simulink library "DAQ_lib_HallPositionTorque"  (R2014b)
settings: Solver=ode45  StartTime=0.0  StopTime=10.0  RelTol=1e-3
undefined symbols (not defined in the file): A_lpf_velocity, ANOMALY_INIT, B1_lpf_velocity, B2_lpf_velocity, Calibration, EnableFT, EncoderAngleLimits, EncoderFiltSys, EncoderThreshold, FTCalibration, GearOffsets, IMUAngleLimits, IMUCommand, IMUThreshold, IMUTorsoOffsets, m_XR17D15x, MAX_ANOMALY, MedullaCommand, MicrostrainFiltSys, MODBUS_TIMEOUT, ResetDAQ, ResetYaw, sample_time, standard, STREAMING_TIMEOUT, TareFT, TorsoCOMOffsets, Ts, TsCAN, TsKVH, UseMicrostrainRate
libraries: xpcethercatlib x207, simulink x53, canmsglib x21, speedgoatlib x13, slrtlib x5, speedgoatlib_IO601 x5, dspswit3 x2, dspmtrx3 x2, xpcseriallib x1, SpeedgoatModified x1
(part 3 of 7)

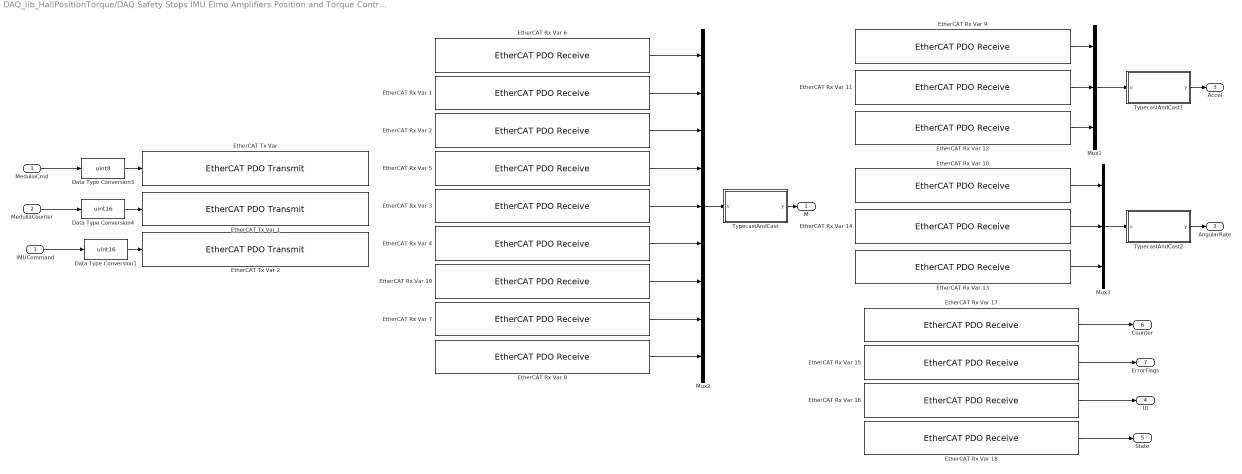
== system DAQ_lib_HallPositionTorque/DAQ Safety Stops IMU Elmo Amplifiers Position and Torque Control with Hall Sensors/DAQ/EtherCATNetwork/EtherCATRobotMicrostrain/IMU_Medulla ==
  MedullaCmd : Inport
  MedullaCounter : Inport  Port=2
  IMUCommand : Inport  Port=3
  Data Type Conversion1 : DataTypeConversion  OutDataTypeStr=uint16  RndMeth=Simplest
  Data Type Conversion3 : DataTypeConversion  OutDataTypeStr=uint8  RndMeth=Simplest
  Data Type Conversion4 : DataTypeConversion  OutDataTypeStr=uint16  RndMeth=Simplest
  EtherCAT Rx Var 1 : xpcethercatlib/EtherCAT PDO Receive  Priority=2  sig_name=Box 7 (ATRIAS 2.1 Microstrain IMU (Medulla 1.5)).M.M12  sig_offset=2784  sig_type=uint32  type_size=32  sig_dim=1  device_id=0  sample_time=0.000500
  EtherCAT Rx Var 10 : xpcethercatlib/EtherCAT PDO Receive  Priority=2  sig_name=Box 7 (ATRIAS 2.1 Microstrain IMU (Medulla 1.5)).Xaxes.XAngRate  sig_offset=2560  sig_type=uint32  type_size=32  sig_dim=1  device_id=0  sample_time=0.000500
  EtherCAT Rx Var 11 : xpcethercatlib/EtherCAT PDO Receive  Priority=2  sig_name=Box 7 (ATRIAS 2.1 Microstrain IMU (Medulla 1.5)).Yaxes.YAccel  sig_offset=2656  sig_type=uint32  type_size=32  sig_dim=1  device_id=0  sample_time=0.000500
  EtherCAT Rx Var 12 : xpcethercatlib/EtherCAT PDO Receive  Priority=2  sig_name=Box 7 (ATRIAS 2.1 Microstrain IMU (Medulla 1.5)).Zaxes.ZAccel  sig_offset=2720  sig_type=uint32  type_size=32  sig_dim=1  device_id=0  sample_time=0.000500
  EtherCAT Rx Var 13 : xpcethercatlib/EtherCAT PDO Receive  Priority=2  sig_name=Box 7 (ATRIAS 2.1 Microstrain IMU (Medulla 1.5)).Zaxes.ZAngRate  sig_offset=2688  sig_type=uint32  type_size=32  sig_dim=1  device_id=0  sample_time=0.000500
  EtherCAT Rx Var 14 : xpcethercatlib/EtherCAT PDO Receive  Priority=2  sig_name=Box 7 (ATRIAS 2.1 Microstrain IMU (Medulla 1.5)).Yaxes.YAngRate  sig_offset=2624  sig_type=uint32  type_size=32  sig_dim=1  device_id=0  sample_time=0.000500
  EtherCAT Rx Var 15 : xpcethercatlib/EtherCAT PDO Receive  Priority=2  sig_name=Box 7 (ATRIAS 2.1 Microstrain IMU (Medulla 1.5)).uController Status.Error Flags  sig_offset=2552  sig_type=uint8  type_size=8  sig_dim=1  device_id=0  sample_time=0.000500
  EtherCAT Rx Var 16 : xpcethercatlib/EtherCAT PDO Receive  Priority=2  sig_name=Box 7 (ATRIAS 2.1 Microstrain IMU (Medulla 1.5)).uController Status.ID  sig_offset=2528  sig_type=uint8  type_size=8  sig_dim=1  device_id=0  sample_time=0.000500
  EtherCAT Rx Var 17 : xpcethercatlib/EtherCAT PDO Receive  Priority=2  sig_name=Box 7 (ATRIAS 2.1 Microstrain IMU (Medulla 1.5)).uController Status.Counter  sig_offset=2544  sig_type=uint8  type_size=8  sig_dim=1  device_id=0  sample_time=0.000500
  EtherCAT Rx Var 18 : xpcethercatlib/EtherCAT PDO Receive  Priority=2  sig_name=Box 7 (ATRIAS 2.1 Microstrain IMU (Medulla 1.5)).uController Status.State  sig_offset=2536  sig_type=uint8  type_size=8  sig_dim=1  device_id=0  sample_time=0.000500
  EtherCAT Rx Var 19 : xpcethercatlib/EtherCAT PDO Receive  Priority=2  sig_name=Box 7 (ATRIAS 2.1 Microstrain IMU (Medulla 1.5)).M.M31  sig_offset=2944  sig_type=uint32  type_size=32  sig_dim=1  device_id=0  sample_time=0.000500
  EtherCAT Rx Var 2 : xpcethercatlib/EtherCAT PDO Receive  Priority=2  sig_name=Box 7 (ATRIAS 2.1 Microstrain IMU (Medulla 1.5)).M.M13  sig_offset=2816  sig_type=uint32  type_size=32  sig_dim=1  device_id=0  sample_time=0.000500
  EtherCAT Rx Var 3 : xpcethercatlib/EtherCAT PDO Receive  Priority=2  sig_name=Box 7 (ATRIAS 2.1 Microstrain IMU (Medulla 1.5)).M.M22  sig_offset=2880  sig_type=uint32  type_size=32  sig_dim=1  device_id=0  sample_time=0.000500
  EtherCAT Rx Var 4 : xpcethercatlib/EtherCAT PDO Receive  Priority=2  sig_name=Box 7 (ATRIAS 2.1 Microstrain IMU (Medulla 1.5)).M.M23  sig_offset=2912  sig_type=uint32  type_size=32  sig_dim=1  device_id=0  sample_time=0.000500
  EtherCAT Rx Var 5 : xpcethercatlib/EtherCAT PDO Receive  Priority=2  sig_name=Box 7 (ATRIAS 2.1 Microstrain IMU (Medulla 1.5)).M.M21  sig_offset=2848  sig_type=uint32  type_size=32  sig_dim=1  device_id=0  sample_time=0.000500
  EtherCAT Rx Var 6 : xpcethercatlib/EtherCAT PDO Receive  Priority=2  sig_name=Box 7 (ATRIAS 2.1 Microstrain IMU (Medulla 1.5)).M.M11  sig_offset=2752  sig_type=uint32  type_size=32  sig_dim=1  device_id=0  sample_time=0.000500
  EtherCAT Rx Var 7 : xpcethercatlib/EtherCAT PDO Receive  Priority=2  sig_name=Box 7 (ATRIAS 2.1 Microstrain IMU (Medulla 1.5)).M.M32  sig_offset=2976  sig_type=uint32  type_size=32  sig_dim=1  device_id=0  sample_time=0.000500
  EtherCAT Rx Var 8 : xpcethercatlib/EtherCAT PDO Receive  Priority=2  sig_name=Box 7 (ATRIAS 2.1 Microstrain IMU (Medulla 1.5)).M.M33  sig_offset=3008  sig_type=uint32  type_size=32  sig_dim=1  device_id=0  sample_time=0.000500
  EtherCAT Rx Var 9 : xpcethercatlib/EtherCAT PDO Receive  Priority=2  sig_name=Box 7 (ATRIAS 2.1 Microstrain IMU (Medulla 1.5)).Xaxes.XAccel  sig_offset=2592  sig_type=uint32  type_size=32  sig_dim=1  device_id=0  sample_time=0.000500
  "EtherCAT Tx Var " : xpcethercatlib/EtherCAT PDO Transmit   Priority=3  sig_name=Box 7 (ATRIAS 2.1 Microstrain IMU (Medulla 1.5)).uControllerInput.Command  sig_offset=2528  sig_type=uint8  type_size=8  sig_dim=1  device_id=0  sample_time=0.000500
  EtherCAT Tx Var 1 : xpcethercatlib/EtherCAT PDO Transmit   Priority=3  sig_name=Box 7 (ATRIAS 2.1 Microstrain IMU (Medulla 1.5)).uControllerInput.Counter  sig_offset=2536  sig_type=uint16  type_size=16  sig_dim=1  device_id=0  sample_time=0.000500
  EtherCAT Tx Var 2 : xpcethercatlib/EtherCAT PDO Transmit   Priority=3  sig_name=Box 7 (ATRIAS 2.1 Microstrain IMU (Medulla 1.5)).uControllerInput.IMU_cmd  sig_offset=2552  sig_type=uint16  type_size=16  sig_dim=1  device_id=0  sample_time=0.000500
  Mux1 : Mux  Inputs=3
  Mux2 : Mux  Inputs=9
  Mux3 : Mux  Inputs=3
  TypecastAndCast : MATLAB Function  TreatAsAtomicUnit=on
  TypecastAndCast1 : MATLAB Function  TreatAsAtomicUnit=on
  TypecastAndCast2 : MATLAB Function  TreatAsAtomicUnit=on
  M : Outport
  AngularRate : Outport  Port=2
  Accel : Outport  Port=3
  ID : Outport  Port=4
  State : Outport  Port=5
  Counter : Outport  Port=6
  ErrorFlags : Outport  Port=7
  wires:
  Data Type Conversion3/1 -> "EtherCAT Tx Var "/1
  Data Type Conversion4/1 -> EtherCAT Tx Var 1/1
  MedullaCmd/1 -> Data Type Conversion3/1
  MedullaCounter/1 -> Data Type Conversion4/1
  IMUCommand/1 -> Data Type Conversion1/1
  Data Type Conversion1/1 -> EtherCAT Tx Var 2/1
  EtherCAT Rx Var 17/1 -> Counter/1
  EtherCAT Rx Var 15/1 -> ErrorFlags/1
  EtherCAT Rx Var 16/1 -> ID/1
  EtherCAT Rx Var 18/1 -> State/1
  EtherCAT Rx Var 13/1 -> Mux3/3
  EtherCAT Rx Var 14/1 -> Mux3/2
  EtherCAT Rx Var 10/1 -> Mux3/1
  EtherCAT Rx Var 12/1 -> Mux1/3
  EtherCAT Rx Var 11/1 -> Mux1/2
  EtherCAT Rx Var 9/1 -> Mux1/1
  Mux1/1 -> TypecastAndCast1/1(u)
  Mux3/1 -> TypecastAndCast2/1(u)
  Mux2/1 -> TypecastAndCast/1(u)
  TypecastAndCast/1(y) -> M/1
  TypecastAndCast1/1(y) -> Accel/1
  TypecastAndCast2/1(y) -> AngularRate/1
  EtherCAT Rx Var 1/1 -> Mux2/2
  EtherCAT Rx Var 19/1 -> Mux2/7
  EtherCAT Rx Var 2/1 -> Mux2/3
  EtherCAT Rx Var 3/1 -> Mux2/5
  EtherCAT Rx Var 4/1 -> Mux2/6
  EtherCAT Rx Var 5/1 -> Mux2/4
  EtherCAT Rx Var 6/1 -> Mux2/1
  EtherCAT Rx Var 7/1 -> Mux2/8
  EtherCAT Rx Var 8/1 -> Mux2/9

== system DAQ_lib_HallPositionTorque/DAQ Safety Stops IMU Elmo Amplifiers Position and Torque Control with Hall Sensors/DAQ/EtherCATNetwork/EtherCATRobotMicrostrain/LegElmo_1L ==
  note: 1, 8 = Position Control
      | 3, 9 = Velocity Control
      | 4, 10 = Current Control
  MedullaCommand : Inport
  Mode of Operation : Inport  Port=2
  Desired Position : Inport  Port=3
  Desired Torque : Inport  Port=4
  Max Torque : Inport  Port=5
  Data Type Conversion{1..2,4,20,42,46} (6 alike) : DataTypeConversion  OutDataTypeStr=double
  Data Type Conversion5 : DataTypeConversion  OutDataTypeStr=int32
  EtherCATSubsystem : Subsystem
  MaxRatedCurrent : Constant  Value=48.47  OutDataTypeStr=double
  State Flow : Stateflow chart  TreatAsAtomicUnit=on
  Subsystem1 : Subsystem
  Subsystem10 : Subsystem
  Subsystem2 : Subsystem
  Subsystem3 : Subsystem
  Subsystem4 : Subsystem
  Subsystem5 : Subsystem
  Subsystem6 : Subsystem
  Subsystem7 : Subsystem
  Terminator : Terminator
  Actual Current : Outport
  Status Word : Outport  Port=2
  Actual Velocity : Outport  Port=3
  Mode of Operation Display : Outport  Port=4
  FaultDetected : Outport  Port=5
  Actual Position : Outport  Port=6
  Control Word Index : Outport  Port=7
  wires:
  Subsystem7/1(ScaledValue) -> EtherCATSubsystem/5(Max Torque)
  Max Torque/1 -> Subsystem7/1(ActualValue)
  [MaxRatedCurrent] -> Subsystem7/2(MaxRatedCurrent)
  Data Type Conversion20/1 -> Actual Current/1
  Data Type Conversion1/1 -> Actual Velocity/1
  Data Type Conversion46/1 -> Mode of Operation Display/1
  Subsystem2/1(SwitchOnDisabledMode) -> State Flow/1(SwitchOnDisabledMode)
  Subsystem3/1(EnabledMode) -> State Flow/2(EnabledMode)
  Subsystem4/1(ReadyToSwitchOnMode) -> State Flow/3(ReadyToSwitchOnMode)
  Subsystem5/1(FaultMode) -> State Flow/4(FaultMode)
  [MaxRatedCurrent] -> Subsystem6/2(MaxRatedCurrent)
  Subsystem6/1(ActualValue) -> Data Type Conversion20/1
  MaxRatedCurrent/1 -> [MaxRatedCurrent]
  State Flow/3(FaultDetected) -> FaultDetected/1
  MedullaCommand/1 -> State Flow/5(MedullaCommand)
  Data Type Conversion2/1 -> Subsystem6/1(ScaledValue)
  Subsystem1/1(ControlWord) -> EtherCATSubsystem/1(Control Word)
  Mode of Operation/1 -> EtherCATSubsystem/2(Mode of Operation)
  EtherCATSubsystem/5(Actual Torque) -> Data Type Conversion2/1
  Data Type Conversion4/1 -> Actual Position/1
  EtherCATSubsystem/2(Mode of Operation Display) -> Data Type Conversion46/1
  EtherCATSubsystem/1(Status Word) -> Subsystem5/1(StatusWord), Subsystem4/1(StatusWord), Subsystem3/1(StatusWord), Subsystem2/1(StatusWord), Data Type Conversion42/1
  Data Type Conversion42/1 -> Status Word/1
  Desired Torque/1 -> Subsystem10/1(ActualValue)
  [MaxRatedCurrent] -> Subsystem10/2(MaxRatedCurrent)
  Subsystem10/1(ScaledValue) -> EtherCATSubsystem/4(Target Torque)
  EtherCATSubsystem/3(Actual Position) -> Data Type Conversion4/1
  EtherCATSubsystem/4(Actual Velocity) -> Data Type Conversion1/1
  State Flow/2(Enable) -> Terminator/1
  Data Type Conversion5/1 -> EtherCATSubsystem/3(Target Position)
  Desired Position/1 -> Data Type Conversion5/1
  State Flow/1(ControlWordIndex) -> Control Word Index/1, Subsystem1/1(ControlWordIndex)

== system DAQ_lib_HallPositionTorque/DAQ Safety Stops IMU Elmo Amplifiers Position and Torque Control with Hall Sensors/DAQ/EtherCATNetwork/EtherCATRobotMicrostrain/LegElmo_1R ==
  note: 1, 8 = Position Control
      | 3, 9 = Velocity Control
      | 4, 10 = Current Control
  MedullaCommand : Inport
  Mode of Operation : Inport  Port=2
  Desired Position : Inport  Port=3
  Desired Torque : Inport  Port=4
  Max Torque : Inport  Port=5
  Data Type Conversion{1..2,4,20,42,46} (6 alike) : DataTypeConversion  OutDataTypeStr=double
  Data Type Conversion5 : DataTypeConversion  OutDataTypeStr=int32
  EtherCATSubsystem : Subsystem
  MaxRatedCurrent : Constant  Value=48.47  OutDataTypeStr=double
  State Flow : Stateflow chart  TreatAsAtomicUnit=on
  Subsystem1 : Subsystem
  Subsystem10 : Subsystem
  Subsystem2 : Subsystem
  Subsystem3 : Subsystem
  Subsystem4 : Subsystem
  Subsystem5 : Subsystem
  Subsystem6 : Subsystem
  Subsystem7 : Subsystem
  Terminator : Terminator
  Actual Current : Outport
  Status Word : Outport  Port=2
  Actual Velocity : Outport  Port=3
  Mode of Operation Display : Outport  Port=4
  FaultDetected : Outport  Port=5
  Actual Position : Outport  Port=6
  Control Word Index : Outport  Port=7
  wires:
  Subsystem7/1(ScaledValue) -> EtherCATSubsystem/5(Max Torque)
  Max Torque/1 -> Subsystem7/1(ActualValue)
  [MaxRatedCurrent] -> Subsystem7/2(MaxRatedCurrent)
  Data Type Conversion20/1 -> Actual Current/1
  Data Type Conversion1/1 -> Actual Velocity/1
  Data Type Conversion46/1 -> Mode of Operation Display/1
  Subsystem2/1(SwitchOnDisabledMode) -> State Flow/1(SwitchOnDisabledMode)
  Subsystem3/1(EnabledMode) -> State Flow/2(EnabledMode)
  Subsystem4/1(ReadyToSwitchOnMode) -> State Flow/3(ReadyToSwitchOnMode)
  Subsystem5/1(FaultMode) -> State Flow/4(FaultMode)
  [MaxRatedCurrent] -> Subsystem6/2(MaxRatedCurrent)
  Subsystem6/1(ActualValue) -> Data Type Conversion20/1
  MaxRatedCurrent/1 -> [MaxRatedCurrent]
  State Flow/3(FaultDetected) -> FaultDetected/1
  MedullaCommand/1 -> State Flow/5(MedullaCommand)
  Data Type Conversion2/1 -> Subsystem6/1(ScaledValue)
  Subsystem1/1(ControlWord) -> EtherCATSubsystem/1(Control Word)
  Mode of Operation/1 -> EtherCATSubsystem/2(Mode of Operation)
  EtherCATSubsystem/5(Actual Torque) -> Data Type Conversion2/1
  Data Type Conversion4/1 -> Actual Position/1
  EtherCATSubsystem/2(Mode of Operation Display) -> Data Type Conversion46/1
  EtherCATSubsystem/1(Status Word) -> Subsystem5/1(StatusWord), Subsystem4/1(StatusWord), Subsystem3/1(StatusWord), Subsystem2/1(StatusWord), Data Type Conversion42/1
  Data Type Conversion42/1 -> Status Word/1
  Desired Torque/1 -> Subsystem10/1(ActualValue)
  [MaxRatedCurrent] -> Subsystem10/2(MaxRatedCurrent)
  Subsystem10/1(ScaledValue) -> EtherCATSubsystem/4(Target Torque)
  EtherCATSubsystem/3(Actual Position) -> Data Type Conversion4/1
  EtherCATSubsystem/4(Actual Velocity) -> Data Type Conversion1/1
  State Flow/2(Enable) -> Terminator/1
  Data Type Conversion5/1 -> EtherCATSubsystem/3(Target Position)
  Desired Position/1 -> Data Type Conversion5/1
  State Flow/1(ControlWordIndex) -> Control Word Index/1, Subsystem1/1(ControlWordIndex)

== system DAQ_lib_HallPositionTorque/DAQ Safety Stops IMU Elmo Amplifiers Position and Torque Control with Hall Sensors/DAQ/EtherCATNetwork/EtherCATRobotMicrostrain/LegElmo_2L ==
  note: 1, 8 = Position Control
      | 3, 9 = Velocity Control
      | 4, 10 = Current Control
  MedullaCommand : Inport
  Mode of Operation : Inport  Port=2
  Desired Position : Inport  Port=3
  Desired Torque : Inport  Port=4
  Max Torque : Inport  Port=5
  Data Type Conversion{1..2,4,20,42,46} (6 alike) : DataTypeConversion  OutDataTypeStr=double
  Data Type Conversion5 : DataTypeConversion  OutDataTypeStr=int32
  EtherCATSubsystem : Subsystem
  MaxRatedCurrent : Constant  Value=48.47  OutDataTypeStr=double
  State Flow : Stateflow chart  TreatAsAtomicUnit=on
  Subsystem1 : Subsystem
  Subsystem10 : Subsystem
  Subsystem2 : Subsystem
  Subsystem3 : Subsystem
  Subsystem4 : Subsystem
  Subsystem5 : Subsystem
  Subsystem6 : Subsystem
  Subsystem7 : Subsystem
  Terminator : Terminator
  Actual Current : Outport
  Status Word : Outport  Port=2
  Actual Velocity : Outport  Port=3
  Mode of Operation Display : Outport  Port=4
  FaultDetected : Outport  Port=5
  Actual Position : Outport  Port=6
  Control Word Index : Outport  Port=7
  wires:
  Subsystem7/1(ScaledValue) -> EtherCATSubsystem/5(Max Torque)
  Max Torque/1 -> Subsystem7/1(ActualValue)
  [MaxRatedCurrent] -> Subsystem7/2(MaxRatedCurrent)
  Data Type Conversion20/1 -> Actual Current/1
  Data Type Conversion1/1 -> Actual Velocity/1
  Data Type Conversion46/1 -> Mode of Operation Display/1
  Subsystem2/1(SwitchOnDisabledMode) -> State Flow/1(SwitchOnDisabledMode)
  Subsystem3/1(EnabledMode) -> State Flow/2(EnabledMode)
  Subsystem4/1(ReadyToSwitchOnMode) -> State Flow/3(ReadyToSwitchOnMode)
  Subsystem5/1(FaultMode) -> State Flow/4(FaultMode)
  [MaxRatedCurrent] -> Subsystem6/2(MaxRatedCurrent)
  Subsystem6/1(ActualValue) -> Data Type Conversion20/1
  MaxRatedCurrent/1 -> [MaxRatedCurrent]
  State Flow/3(FaultDetected) -> FaultDetected/1
  MedullaCommand/1 -> State Flow/5(MedullaCommand)
  Data Type Conversion2/1 -> Subsystem6/1(ScaledValue)
  Subsystem1/1(ControlWord) -> EtherCATSubsystem/1(Control Word)
  Mode of Operation/1 -> EtherCATSubsystem/2(Mode of Operation)
  EtherCATSubsystem/5(Actual Torque) -> Data Type Conversion2/1
  Data Type Conversion4/1 -> Actual Position/1
  EtherCATSubsystem/2(Mode of Operation Display) -> Data Type Conversion46/1
  EtherCATSubsystem/1(Status Word) -> Subsystem5/1(StatusWord), Subsystem4/1(StatusWord), Subsystem3/1(StatusWord), Subsystem2/1(StatusWord), Data Type Conversion42/1
  Data Type Conversion42/1 -> Status Word/1
  Desired Torque/1 -> Subsystem10/1(ActualValue)
  [MaxRatedCurrent] -> Subsystem10/2(MaxRatedCurrent)
  Subsystem10/1(ScaledValue) -> EtherCATSubsystem/4(Target Torque)
  EtherCATSubsystem/3(Actual Position) -> Data Type Conversion4/1
  EtherCATSubsystem/4(Actual Velocity) -> Data Type Conversion1/1
  State Flow/2(Enable) -> Terminator/1
  Data Type Conversion5/1 -> EtherCATSubsystem/3(Target Position)
  Desired Position/1 -> Data Type Conversion5/1
  State Flow/1(ControlWordIndex) -> Control Word Index/1, Subsystem1/1(ControlWordIndex)

== system DAQ_lib_HallPositionTorque/DAQ Safety Stops IMU Elmo Amplifiers Position and Torque Control with Hall Sensors/DAQ/EtherCATNetwork/EtherCATRobotMicrostrain/LegElmo_2R ==
  note: 1, 8 = Position Control
      | 3, 9 = Velocity Control
      | 4, 10 = Current Control
  MedullaCommand : Inport
  Mode of Operation : Inport  Port=2
  Desired Position : Inport  Port=3
  Desired Torque : Inport  Port=4
  Max Torque : Inport  Port=5
  Data Type Conversion{1..2,4,20,42,46} (6 alike) : DataTypeConversion  OutDataTypeStr=double
  Data Type Conversion5 : DataTypeConversion  OutDataTypeStr=int32
  EtherCATSubsystem : Subsystem
  MaxRatedCurrent : Constant  Value=48.47  OutDataTypeStr=double
  State Flow : Stateflow chart  TreatAsAtomicUnit=on
  Subsystem1 : Subsystem
  Subsystem10 : Subsystem
  Subsystem2 : Subsystem
  Subsystem3 : Subsystem
  Subsystem4 : Subsystem
  Subsystem5 : Subsystem
  Subsystem6 : Subsystem
  Subsystem7 : Subsystem
  Terminator : Terminator
  Actual Current : Outport
  Status Word : Outport  Port=2
  Actual Velocity : Outport  Port=3
  Mode of Operation Display : Outport  Port=4
  FaultDetected : Outport  Port=5
  Actual Position : Outport  Port=6
  Control Word Index : Outport  Port=7
  wires:
  Subsystem7/1(ScaledValue) -> EtherCATSubsystem/5(Max Torque)
  Max Torque/1 -> Subsystem7/1(ActualValue)
  [MaxRatedCurrent] -> Subsystem7/2(MaxRatedCurrent)
  Data Type Conversion20/1 -> Actual Current/1
  Data Type Conversion1/1 -> Actual Velocity/1
  Data Type Conversion46/1 -> Mode of Operation Display/1
  Subsystem2/1(SwitchOnDisabledMode) -> State Flow/1(SwitchOnDisabledMode)
  Subsystem3/1(EnabledMode) -> State Flow/2(EnabledMode)
  Subsystem4/1(ReadyToSwitchOnMode) -> State Flow/3(ReadyToSwitchOnMode)
  Subsystem5/1(FaultMode) -> State Flow/4(FaultMode)
  [MaxRatedCurrent] -> Subsystem6/2(MaxRatedCurrent)
  Subsystem6/1(ActualValue) -> Data Type Conversion20/1
  MaxRatedCurrent/1 -> [MaxRatedCurrent]
  State Flow/3(FaultDetected) -> FaultDetected/1
  MedullaCommand/1 -> State Flow/5(MedullaCommand)
  Data Type Conversion2/1 -> Subsystem6/1(ScaledValue)
  Subsystem1/1(ControlWord) -> EtherCATSubsystem/1(Control Word)
  Mode of Operation/1 -> EtherCATSubsystem/2(Mode of Operation)
  EtherCATSubsystem/5(Actual Torque) -> Data Type Conversion2/1
  Data Type Conversion4/1 -> Actual Position/1
  EtherCATSubsystem/2(Mode of Operation Display) -> Data Type Conversion46/1
  EtherCATSubsystem/1(Status Word) -> Subsystem5/1(StatusWord), Subsystem4/1(StatusWord), Subsystem3/1(StatusWord), Subsystem2/1(StatusWord), Data Type Conversion42/1
  Data Type Conversion42/1 -> Status Word/1
  Desired Torque/1 -> Subsystem10/1(ActualValue)
  [MaxRatedCurrent] -> Subsystem10/2(MaxRatedCurrent)
  Subsystem10/1(ScaledValue) -> EtherCATSubsystem/4(Target Torque)
  EtherCATSubsystem/3(Actual Position) -> Data Type Conversion4/1
  EtherCATSubsystem/4(Actual Velocity) -> Data Type Conversion1/1
  State Flow/2(Enable) -> Terminator/1
  Data Type Conversion5/1 -> EtherCATSubsystem/3(Target Position)
  Desired Position/1 -> Data Type Conversion5/1
  State Flow/1(ControlWordIndex) -> Control Word Index/1, Subsystem1/1(ControlWordIndex)

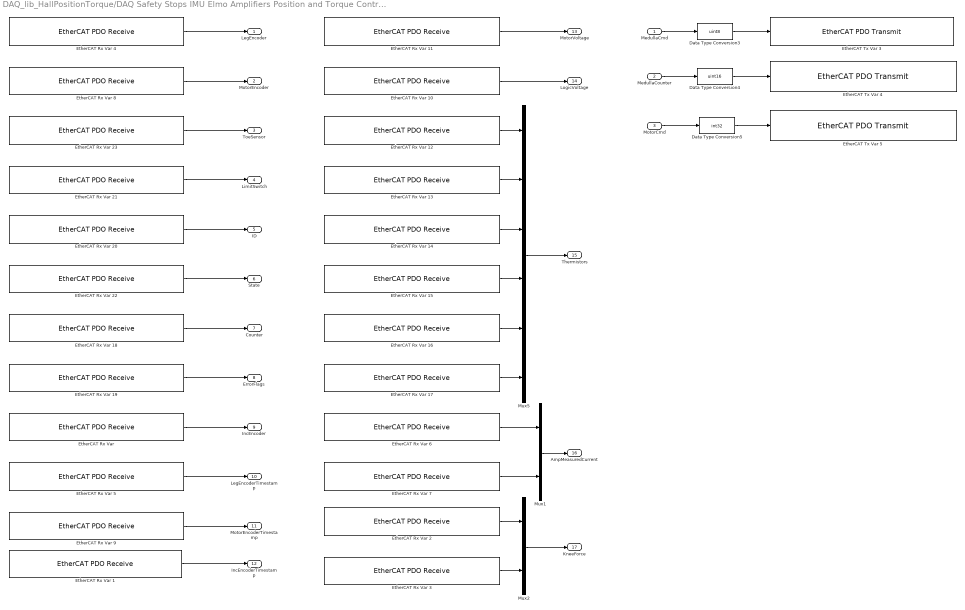
== system DAQ_lib_HallPositionTorque/DAQ Safety Stops IMU Elmo Amplifiers Position and Torque Control with Hall Sensors/DAQ/EtherCATNetwork/EtherCATRobotMicrostrain/LegMedulla_1L ==
  MedullaCmd : Inport
  MedullaCounter : Inport  Port=2
  MotorCmd : Inport  Port=3
  Data Type Conversion3 : DataTypeConversion  OutDataTypeStr=uint8  RndMeth=Simplest
  Data Type Conversion4 : DataTypeConversion  OutDataTypeStr=uint16  RndMeth=Simplest
  Data Type Conversion5 : DataTypeConversion  OutDataTypeStr=int32  RndMeth=Simplest
  "EtherCAT Rx Var " : xpcethercatlib/EtherCAT PDO Receive  Priority=2  sig_name=Box 1 (ATRIAS 2.1 Leg (Medulla 1.5)).Incremental Encoder.Incremental Encoder  sig_offset=744  sig_type=uint16  type_size=16  sig_dim=1  device_id=0  sample_time=0.000500
  EtherCAT Rx Var 1 : xpcethercatlib/EtherCAT PDO Receive  Priority=2  sig_name=Box 1 (ATRIAS 2.1 Leg (Medulla 1.5)).Incremental Encoder.Incremental Encoder Timestamp  sig_offset=760  sig_type=uint16  type_size=16  sig_dim=1  device_id=0  sample_time=0.000500
  EtherCAT Rx Var 10 : xpcethercatlib/EtherCAT PDO Receive  Priority=2  sig_name=Box 1 (ATRIAS 2.1 Leg (Medulla 1.5)).Power.Logic Voltage  sig_offset=792  sig_type=uint16  type_size=16  sig_dim=1  device_id=0  sample_time=0.000500
  EtherCAT Rx Var 11 : xpcethercatlib/EtherCAT PDO Receive  Priority=2  sig_name=Box 1 (ATRIAS 2.1 Leg (Medulla 1.5)).Power.Motor Voltage  sig_offset=776  sig_type=uint16  type_size=16  sig_dim=1  device_id=0  sample_time=0.000500
  EtherCAT Rx Var 12 : xpcethercatlib/EtherCAT PDO Receive  Priority=2  sig_name=Box 1 (ATRIAS 2.1 Leg (Medulla 1.5)).Thermistors.Thermistor 0  sig_offset=808  sig_type=uint16  type_size=16  sig_dim=1  device_id=0  sample_time=0.000500
  EtherCAT Rx Var 13 : xpcethercatlib/EtherCAT PDO Receive  Priority=2  sig_name=Box 1 (ATRIAS 2.1 Leg (Medulla 1.5)).Thermistors.Thermistor 1  sig_offset=824  sig_type=uint16  type_size=16  sig_dim=1  device_id=0  sample_time=0.000500
  EtherCAT Rx Var 14 : xpcethercatlib/EtherCAT PDO Receive  Priority=2  sig_name=Box 1 (ATRIAS 2.1 Leg (Medulla 1.5)).Thermistors.Thermistor 2  sig_offset=840  sig_type=uint16  type_size=16  sig_dim=1  device_id=0  sample_time=0.000500
  EtherCAT Rx Var 15 : xpcethercatlib/EtherCAT PDO Receive  Priority=2  sig_name=Box 1 (ATRIAS 2.1 Leg (Medulla 1.5)).Thermistors.Thermistor 3  sig_offset=856  sig_type=uint16  type_size=16  sig_dim=1  device_id=0  sample_time=0.000500
  EtherCAT Rx Var 16 : xpcethercatlib/EtherCAT PDO Receive  Priority=2  sig_name=Box 1 (ATRIAS 2.1 Leg (Medulla 1.5)).Thermistors.Thermistor 4  sig_offset=872  sig_type=uint16  type_size=16  sig_dim=1  device_id=0  sample_time=0.000500
  EtherCAT Rx Var 17 : xpcethercatlib/EtherCAT PDO Receive  Priority=2  sig_name=Box 1 (ATRIAS 2.1 Leg (Medulla 1.5)).Thermistors.Thermistor 5  sig_offset=888  sig_type=uint16  type_size=16  sig_dim=1  device_id=0  sample_time=0.000500
  EtherCAT Rx Var 18 : xpcethercatlib/EtherCAT PDO Receive  Priority=2  sig_name=Box 1 (ATRIAS 2.1 Leg (Medulla 1.5)).uController Status.Counter  sig_offset=608  sig_type=uint8  type_size=8  sig_dim=1  device_id=0  sample_time=0.000500
  EtherCAT Rx Var 19 : xpcethercatlib/EtherCAT PDO Receive  Priority=2  sig_name=Box 1 (ATRIAS 2.1 Leg (Medulla 1.5)).uController Status.Error Flags  sig_offset=616  sig_type=uint8  type_size=8  sig_dim=1  device_id=0  sample_time=0.000500
  EtherCAT Rx Var 2 : xpcethercatlib/EtherCAT PDO Receive  Priority=2  sig_name=Box 1 (ATRIAS 2.1 Leg (Medulla 1.5)).Knee Force.Knee Force 1  sig_offset=936  sig_type=uint16  type_size=16  sig_dim=1  device_id=0  sample_time=0.000500
  EtherCAT Rx Var 20 : xpcethercatlib/EtherCAT PDO Receive  Priority=2  sig_name=Box 1 (ATRIAS 2.1 Leg (Medulla 1.5)).uController Status.ID  sig_offset=592  sig_type=uint8  type_size=8  sig_dim=1  device_id=0  sample_time=0.000500
  EtherCAT Rx Var 21 : xpcethercatlib/EtherCAT PDO Receive  Priority=2  sig_name=Box 1 (ATRIAS 2.1 Leg (Medulla 1.5)).uController Status.Limit Switch  sig_offset=624  sig_type=uint8  type_size=8  sig_dim=1  device_id=0  sample_time=0.000500
  EtherCAT Rx Var 22 : xpcethercatlib/EtherCAT PDO Receive  Priority=2  sig_name=Box 1 (ATRIAS 2.1 Leg (Medulla 1.5)).uController Status.State  sig_offset=600  sig_type=uint8  type_size=8  sig_dim=1  device_id=0  sample_time=0.000500
  EtherCAT Rx Var 23 : xpcethercatlib/EtherCAT PDO Receive  Priority=2  sig_name=Box 1 (ATRIAS 2.1 Leg (Medulla 1.5)).uController Status.Toe Sensor  sig_offset=632  sig_type=uint16  type_size=16  sig_dim=1  device_id=0  sample_time=0.000500
  EtherCAT Rx Var 3 : xpcethercatlib/EtherCAT PDO Receive  Priority=2  sig_name=Box 1 (ATRIAS 2.1 Leg (Medulla 1.5)).Knee Force.Knee Force 2  sig_offset=952  sig_type=uint16  type_size=16  sig_dim=1  device_id=0  sample_time=0.000500
  EtherCAT Rx Var 4 : xpcethercatlib/EtherCAT PDO Receive  Priority=2  sig_name=Box 1 (ATRIAS 2.1 Leg (Medulla 1.5)).Leg Encoder.Leg Encoder  sig_offset=696  sig_type=uint32  type_size=32  sig_dim=1  device_id=0  sample_time=0.000500
  EtherCAT Rx Var 5 : xpcethercatlib/EtherCAT PDO Receive  Priority=2  sig_name=Box 1 (ATRIAS 2.1 Leg (Medulla 1.5)).Leg Encoder.Leg Encoder Timestamp  sig_offset=728  sig_type=uint16  type_size=16  sig_dim=1  device_id=0  sample_time=0.000500
  EtherCAT Rx Var 6 : xpcethercatlib/EtherCAT PDO Receive  Priority=2  sig_name=Box 1 (ATRIAS 2.1 Leg (Medulla 1.5)).Measured Current.Amp 1 Measured Current  sig_offset=904  sig_type=int16  type_size=16  sig_dim=1  device_id=0  sample_time=0.000500
  EtherCAT Rx Var 7 : xpcethercatlib/EtherCAT PDO Receive  Priority=2  sig_name=Box 1 (ATRIAS 2.1 Leg (Medulla 1.5)).Measured Current.Amp 2 Measured Current  sig_offset=920  sig_type=int16  type_size=16  sig_dim=1  device_id=0  sample_time=0.000500
  EtherCAT Rx Var 8 : xpcethercatlib/EtherCAT PDO Receive  Priority=2  sig_name=Box 1 (ATRIAS 2.1 Leg (Medulla 1.5)).Motor Encoder.Motor Encoder  sig_offset=648  sig_type=uint32  type_size=32  sig_dim=1  device_id=0  sample_time=0.000500
  EtherCAT Rx Var 9 : xpcethercatlib/EtherCAT PDO Receive  Priority=2  sig_name=Box 1 (ATRIAS 2.1 Leg (Medulla 1.5)).Motor Encoder.Motor Encoder Timestamp  sig_offset=680  sig_type=uint16  type_size=16  sig_dim=1  device_id=0  sample_time=0.000500
  EtherCAT Tx Var 3 : xpcethercatlib/EtherCAT PDO Transmit   Priority=3  sig_name=Box 1 (ATRIAS 2.1 Leg (Medulla 1.5)).uControllerInput.Command  sig_offset=592  sig_type=uint8  type_size=8  sig_dim=1  device_id=0  sample_time=0.000500
  EtherCAT Tx Var 4 : xpcethercatlib/EtherCAT PDO Transmit   Priority=3  sig_name=Box 1 (ATRIAS 2.1 Leg (Medulla 1.5)).uControllerInput.Counter  sig_offset=600  sig_type=uint16  type_size=16  sig_dim=1  device_id=0  sample_time=0.000500
  EtherCAT Tx Var 5 : xpcethercatlib/EtherCAT PDO Transmit   Priority=3  sig_name=Box 1 (ATRIAS 2.1 Leg (Medulla 1.5)).uControllerInput.Motor Current  sig_offset=616  sig_type=int32  type_size=32  sig_dim=1  device_id=0  sample_time=0.000500
  Mux1 : Mux  Inputs=2
  Mux2 : Mux  Inputs=2
  Mux5 : Mux  Inputs=6
  LegEncoder : Outport
  MotorEncoder : Outport  Port=2
  ToeSensor : Outport  Port=3
  LimitSwitch : Outport  Port=4
  ID : Outport  Port=5
  State : Outport  Port=6
  Counter : Outport  Port=7
  ErrorFlags : Outport  Port=8
  IncEncoder : Outport  Port=9
  LegEncoderTimestamp : Outport  Port=10
  MotorEncoderTimestamp : Outport  Port=11
  IncEncoderTimestamp : Outport  Port=12
  MotorVoltage : Outport  Port=13
  LogicVoltage : Outport  Port=14
  Thermistors : Outport  Port=15
  AmpMeasuredCurrent : Outport  Port=16
  KneeForce : Outport  Port=17
  wires:
  Data Type Conversion3/1 -> EtherCAT Tx Var 3/1
  Data Type Conversion4/1 -> EtherCAT Tx Var 4/1
  Data Type Conversion5/1 -> EtherCAT Tx Var 5/1
  "EtherCAT Rx Var "/1 -> IncEncoder/1
  EtherCAT Rx Var 1/1 -> IncEncoderTimestamp/1
  EtherCAT Rx Var 2/1 -> Mux2/1
  EtherCAT Rx Var 4/1 -> LegEncoder/1
  EtherCAT Rx Var 5/1 -> LegEncoderTimestamp/1
  EtherCAT Rx Var 6/1 -> Mux1/1
  EtherCAT Rx Var 8/1 -> MotorEncoder/1
  EtherCAT Rx Var 9/1 -> MotorEncoderTimestamp/1
  EtherCAT Rx Var 10/1 -> LogicVoltage/1
  EtherCAT Rx Var 11/1 -> MotorVoltage/1
  EtherCAT Rx Var 13/1 -> Mux5/2
  EtherCAT Rx Var 14/1 -> Mux5/3
  EtherCAT Rx Var 15/1 -> Mux5/4
  EtherCAT Rx Var 16/1 -> Mux5/5
  EtherCAT Rx Var 17/1 -> Mux5/6
  EtherCAT Rx Var 18/1 -> Counter/1
  EtherCAT Rx Var 19/1 -> ErrorFlags/1
  EtherCAT Rx Var 20/1 -> ID/1
  EtherCAT Rx Var 21/1 -> LimitSwitch/1
  EtherCAT Rx Var 22/1 -> State/1
  EtherCAT Rx Var 23/1 -> ToeSensor/1
  MedullaCmd/1 -> Data Type Conversion3/1
  MedullaCounter/1 -> Data Type Conversion4/1
  MotorCmd/1 -> Data Type Conversion5/1
  EtherCAT Rx Var 12/1 -> Mux5/1
  Mux5/1 -> Thermistors/1
  Mux1/1 -> AmpMeasuredCurrent/1
  EtherCAT Rx Var 7/1 -> Mux1/2
  EtherCAT Rx Var 3/1 -> Mux2/2
  Mux2/1 -> KneeForce/1

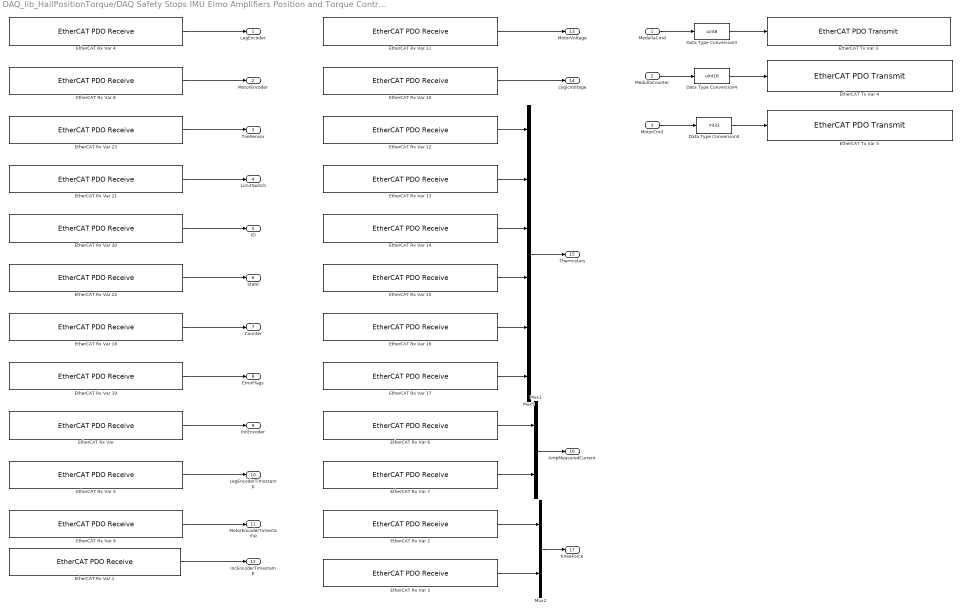
== system DAQ_lib_HallPositionTorque/DAQ Safety Stops IMU Elmo Amplifiers Position and Torque Control with Hall Sensors/DAQ/EtherCATNetwork/EtherCATRobotMicrostrain/LegMedulla_1R ==
  MedullaCmd : Inport
  MedullaCounter : Inport  Port=2
  MotorCmd : Inport  Port=3
  Data Type Conversion3 : DataTypeConversion  OutDataTypeStr=uint8  RndMeth=Simplest
  Data Type Conversion4 : DataTypeConversion  OutDataTypeStr=uint16  RndMeth=Simplest
  Data Type Conversion5 : DataTypeConversion  OutDataTypeStr=int32  RndMeth=Simplest
  "EtherCAT Rx Var " : xpcethercatlib/EtherCAT PDO Receive  Priority=2  sig_name=Box 3 (ATRIAS 2.1 Leg (Medulla 1.5)).Incremental Encoder.Incremental Encoder  sig_offset=1496  sig_type=uint16  type_size=16  sig_dim=1  device_id=0  sample_time=0.000500
  EtherCAT Rx Var 1 : xpcethercatlib/EtherCAT PDO Receive  Priority=2  sig_name=Box 3 (ATRIAS 2.1 Leg (Medulla 1.5)).Incremental Encoder.Incremental Encoder Timestamp  sig_offset=1512  sig_type=uint16  type_size=16  sig_dim=1  device_id=0  sample_time=0.000500
  EtherCAT Rx Var 10 : xpcethercatlib/EtherCAT PDO Receive  Priority=2  sig_name=Box 3 (ATRIAS 2.1 Leg (Medulla 1.5)).Power.Logic Voltage  sig_offset=1544  sig_type=uint16  type_size=16  sig_dim=1  device_id=0  sample_time=0.000500
  EtherCAT Rx Var 11 : xpcethercatlib/EtherCAT PDO Receive  Priority=2  sig_name=Box 3 (ATRIAS 2.1 Leg (Medulla 1.5)).Power.Motor Voltage  sig_offset=1528  sig_type=uint16  type_size=16  sig_dim=1  device_id=0  sample_time=0.000500
  EtherCAT Rx Var 12 : xpcethercatlib/EtherCAT PDO Receive  Priority=2  sig_name=Box 3 (ATRIAS 2.1 Leg (Medulla 1.5)).Thermistors.Thermistor 0  sig_offset=1560  sig_type=uint16  type_size=16  sig_dim=1  device_id=0  sample_time=0.000500
  EtherCAT Rx Var 13 : xpcethercatlib/EtherCAT PDO Receive  Priority=2  sig_name=Box 3 (ATRIAS 2.1 Leg (Medulla 1.5)).Thermistors.Thermistor 1  sig_offset=1576  sig_type=uint16  type_size=16  sig_dim=1  device_id=0  sample_time=0.000500
  EtherCAT Rx Var 14 : xpcethercatlib/EtherCAT PDO Receive  Priority=2  sig_name=Box 3 (ATRIAS 2.1 Leg (Medulla 1.5)).Thermistors.Thermistor 2  sig_offset=1592  sig_type=uint16  type_size=16  sig_dim=1  device_id=0  sample_time=0.000500
  EtherCAT Rx Var 15 : xpcethercatlib/EtherCAT PDO Receive  Priority=2  sig_name=Box 3 (ATRIAS 2.1 Leg (Medulla 1.5)).Thermistors.Thermistor 3  sig_offset=1608  sig_type=uint16  type_size=16  sig_dim=1  device_id=0  sample_time=0.000500
  EtherCAT Rx Var 16 : xpcethercatlib/EtherCAT PDO Receive  Priority=2  sig_name=Box 3 (ATRIAS 2.1 Leg (Medulla 1.5)).Thermistors.Thermistor 4  sig_offset=1624  sig_type=uint16  type_size=16  sig_dim=1  device_id=0  sample_time=0.000500
  EtherCAT Rx Var 17 : xpcethercatlib/EtherCAT PDO Receive  Priority=2  sig_name=Box 3 (ATRIAS 2.1 Leg (Medulla 1.5)).Thermistors.Thermistor 5  sig_offset=1640  sig_type=uint16  type_size=16  sig_dim=1  device_id=0  sample_time=0.000500
  EtherCAT Rx Var 18 : xpcethercatlib/EtherCAT PDO Receive  Priority=2  sig_name=Box 3 (ATRIAS 2.1 Leg (Medulla 1.5)).uController Status.Counter  sig_offset=1360  sig_type=uint8  type_size=8  sig_dim=1  device_id=0  sample_time=0.000500
  EtherCAT Rx Var 19 : xpcethercatlib/EtherCAT PDO Receive  Priority=2  sig_name=Box 3 (ATRIAS 2.1 Leg (Medulla 1.5)).uController Status.Error Flags  sig_offset=1368  sig_type=uint8  type_size=8  sig_dim=1  device_id=0  sample_time=0.000500
  EtherCAT Rx Var 2 : xpcethercatlib/EtherCAT PDO Receive  Priority=2  sig_name=Box 3 (ATRIAS 2.1 Leg (Medulla 1.5)).Knee Force.Knee Force 1  sig_offset=1688  sig_type=uint16  type_size=16  sig_dim=1  device_id=0  sample_time=0.000500
  EtherCAT Rx Var 20 : xpcethercatlib/EtherCAT PDO Receive  Priority=2  sig_name=Box 3 (ATRIAS 2.1 Leg (Medulla 1.5)).uController Status.ID  sig_offset=1344  sig_type=uint8  type_size=8  sig_dim=1  device_id=0  sample_time=0.000500
  EtherCAT Rx Var 21 : xpcethercatlib/EtherCAT PDO Receive  Priority=2  sig_name=Box 3 (ATRIAS 2.1 Leg (Medulla 1.5)).uController Status.Limit Switch  sig_offset=1376  sig_type=uint8  type_size=8  sig_dim=1  device_id=0  sample_time=0.000500
  EtherCAT Rx Var 22 : xpcethercatlib/EtherCAT PDO Receive  Priority=2  sig_name=Box 3 (ATRIAS 2.1 Leg (Medulla 1.5)).uController Status.State  sig_offset=1352  sig_type=uint8  type_size=8  sig_dim=1  device_id=0  sample_time=0.000500
  EtherCAT Rx Var 23 : xpcethercatlib/EtherCAT PDO Receive  Priority=2  sig_name=Box 3 (ATRIAS 2.1 Leg (Medulla 1.5)).uController Status.Toe Sensor  sig_offset=1384  sig_type=uint16  type_size=16  sig_dim=1  device_id=0  sample_time=0.000500
  EtherCAT Rx Var 3 : xpcethercatlib/EtherCAT PDO Receive  Priority=2  sig_name=Box 3 (ATRIAS 2.1 Leg (Medulla 1.5)).Knee Force.Knee Force 2  sig_offset=1704  sig_type=uint16  type_size=16  sig_dim=1  device_id=0  sample_time=0.000500
  EtherCAT Rx Var 4 : xpcethercatlib/EtherCAT PDO Receive  Priority=2  sig_name=Box 3 (ATRIAS 2.1 Leg (Medulla 1.5)).Leg Encoder.Leg Encoder  sig_offset=1448  sig_type=uint32  type_size=32  sig_dim=1  device_id=0  sample_time=0.000500
  EtherCAT Rx Var 5 : xpcethercatlib/EtherCAT PDO Receive  Priority=2  sig_name=Box 3 (ATRIAS 2.1 Leg (Medulla 1.5)).Leg Encoder.Leg Encoder Timestamp  sig_offset=1480  sig_type=uint16  type_size=16  sig_dim=1  device_id=0  sample_time=0.000500
  EtherCAT Rx Var 6 : xpcethercatlib/EtherCAT PDO Receive  Priority=2  sig_name=Box 3 (ATRIAS 2.1 Leg (Medulla 1.5)).Measured Current.Amp 1 Measured Current  sig_offset=1656  sig_type=int16  type_size=16  sig_dim=1  device_id=0  sample_time=0.000500
  EtherCAT Rx Var 7 : xpcethercatlib/EtherCAT PDO Receive  Priority=2  sig_name=Box 3 (ATRIAS 2.1 Leg (Medulla 1.5)).Measured Current.Amp 2 Measured Current  sig_offset=1672  sig_type=int16  type_size=16  sig_dim=1  device_id=0  sample_time=0.000500
  EtherCAT Rx Var 8 : xpcethercatlib/EtherCAT PDO Receive  Priority=2  sig_name=Box 3 (ATRIAS 2.1 Leg (Medulla 1.5)).Motor Encoder.Motor Encoder  sig_offset=1400  sig_type=uint32  type_size=32  sig_dim=1  device_id=0  sample_time=0.000500
  EtherCAT Rx Var 9 : xpcethercatlib/EtherCAT PDO Receive  Priority=2  sig_name=Box 3 (ATRIAS 2.1 Leg (Medulla 1.5)).Motor Encoder.Motor Encoder Timestamp  sig_offset=1432  sig_type=uint16  type_size=16  sig_dim=1  device_id=0  sample_time=0.000500
  EtherCAT Tx Var 3 : xpcethercatlib/EtherCAT PDO Transmit   Priority=3  sig_name=Box 3 (ATRIAS 2.1 Leg (Medulla 1.5)).uControllerInput.Command  sig_offset=1344  sig_type=uint8  type_size=8  sig_dim=1  device_id=0  sample_time=0.000500
  EtherCAT Tx Var 4 : xpcethercatlib/EtherCAT PDO Transmit   Priority=3  sig_name=Box 3 (ATRIAS 2.1 Leg (Medulla 1.5)).uControllerInput.Counter  sig_offset=1352  sig_type=uint16  type_size=16  sig_dim=1  device_id=0  sample_time=0.000500
  EtherCAT Tx Var 5 : xpcethercatlib/EtherCAT PDO Transmit   Priority=3  sig_name=Box 3 (ATRIAS 2.1 Leg (Medulla 1.5)).uControllerInput.Motor Current  sig_offset=1368  sig_type=int32  type_size=32  sig_dim=1  device_id=0  sample_time=0.000500
  Mux1 : Mux  Inputs=2
  Mux2 : Mux  Inputs=2
  Mux5 : Mux  Inputs=6
  LegEncoder : Outport
  MotorEncoder : Outport  Port=2
  ToeSensor : Outport  Port=3
  LimitSwitch : Outport  Port=4
  ID : Outport  Port=5
  State : Outport  Port=6
  Counter : Outport  Port=7
  ErrorFlags : Outport  Port=8
  IncEncoder : Outport  Port=9
  LegEncoderTimestamp : Outport  Port=10
  MotorEncoderTimestamp : Outport  Port=11
  IncEncoderTimestamp : Outport  Port=12
  MotorVoltage : Outport  Port=13
  LogicVoltage : Outport  Port=14
  Thermistors : Outport  Port=15
  AmpMeasuredCurrent : Outport  Port=16
  KneeForce : Outport  Port=17
  wires:
  Data Type Conversion3/1 -> EtherCAT Tx Var 3/1
  Data Type Conversion4/1 -> EtherCAT Tx Var 4/1
  Data Type Conversion5/1 -> EtherCAT Tx Var 5/1
  "EtherCAT Rx Var "/1 -> IncEncoder/1
  EtherCAT Rx Var 1/1 -> IncEncoderTimestamp/1
  EtherCAT Rx Var 2/1 -> Mux2/1
  EtherCAT Rx Var 3/1 -> Mux2/2
  EtherCAT Rx Var 4/1 -> LegEncoder/1
  EtherCAT Rx Var 5/1 -> LegEncoderTimestamp/1
  EtherCAT Rx Var 6/1 -> Mux1/1
  EtherCAT Rx Var 7/1 -> Mux1/2
  EtherCAT Rx Var 8/1 -> MotorEncoder/1
  EtherCAT Rx Var 9/1 -> MotorEncoderTimestamp/1
  EtherCAT Rx Var 10/1 -> LogicVoltage/1
  EtherCAT Rx Var 11/1 -> MotorVoltage/1
  EtherCAT Rx Var 12/1 -> Mux5/1
  EtherCAT Rx Var 13/1 -> Mux5/2
  EtherCAT Rx Var 14/1 -> Mux5/3
  EtherCAT Rx Var 15/1 -> Mux5/4
  EtherCAT Rx Var 16/1 -> Mux5/5
  EtherCAT Rx Var 17/1 -> Mux5/6
  EtherCAT Rx Var 18/1 -> Counter/1
  EtherCAT Rx Var 19/1 -> ErrorFlags/1
  EtherCAT Rx Var 20/1 -> ID/1
  EtherCAT Rx Var 21/1 -> LimitSwitch/1
  EtherCAT Rx Var 22/1 -> State/1
  EtherCAT Rx Var 23/1 -> ToeSensor/1
  MedullaCmd/1 -> Data Type Conversion3/1
  MedullaCounter/1 -> Data Type Conversion4/1
  MotorCmd/1 -> Data Type Conversion5/1
  Mux5/1 -> Thermistors/1
  Mux1/1 -> AmpMeasuredCurrent/1
  Mux2/1 -> KneeForce/1

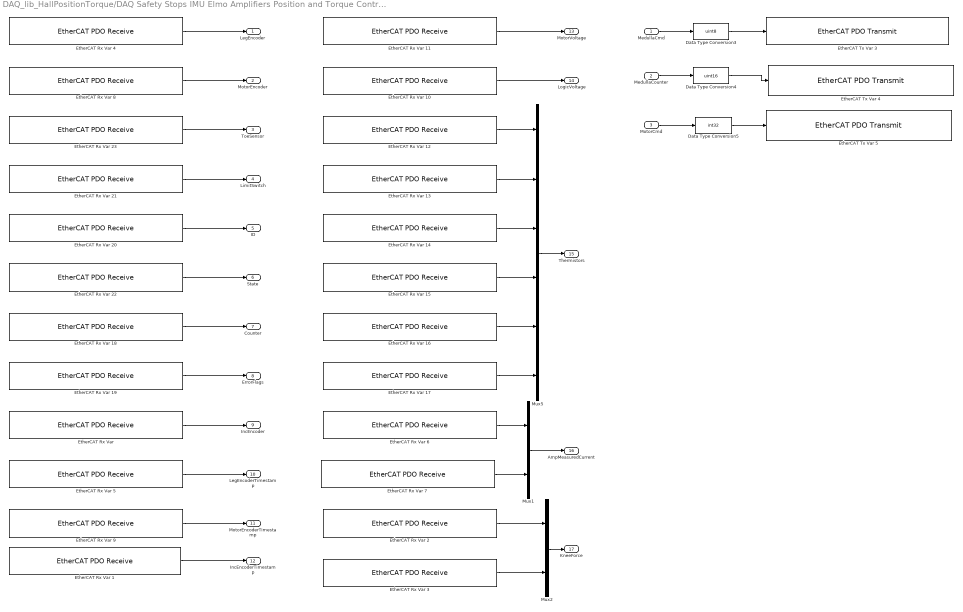
== system DAQ_lib_HallPositionTorque/DAQ Safety Stops IMU Elmo Amplifiers Position and Torque Control with Hall Sensors/DAQ/EtherCATNetwork/EtherCATRobotMicrostrain/LegMedulla_2L ==
  MedullaCmd : Inport
  MedullaCounter : Inport  Port=2
  MotorCmd : Inport  Port=3
  Data Type Conversion3 : DataTypeConversion  OutDataTypeStr=uint8  RndMeth=Simplest
  Data Type Conversion4 : DataTypeConversion  OutDataTypeStr=uint16  RndMeth=Simplest
  Data Type Conversion5 : DataTypeConversion  OutDataTypeStr=int32  RndMeth=Simplest
  "EtherCAT Rx Var " : xpcethercatlib/EtherCAT PDO Receive  Priority=2  sig_name=Box 2 (ATRIAS 2.1 Leg (Medulla 1.5)).Incremental Encoder.Incremental Encoder  sig_offset=1120  sig_type=uint16  type_size=16  sig_dim=1  device_id=0  sample_time=0.000500
  EtherCAT Rx Var 1 : xpcethercatlib/EtherCAT PDO Receive  Priority=2  sig_name=Box 2 (ATRIAS 2.1 Leg (Medulla 1.5)).Incremental Encoder.Incremental Encoder Timestamp  sig_offset=1136  sig_type=uint16  type_size=16  sig_dim=1  device_id=0  sample_time=0.000500
  EtherCAT Rx Var 10 : xpcethercatlib/EtherCAT PDO Receive  Priority=2  sig_name=Box 2 (ATRIAS 2.1 Leg (Medulla 1.5)).Power.Logic Voltage  sig_offset=1168  sig_type=uint16  type_size=16  sig_dim=1  device_id=0  sample_time=0.000500
  EtherCAT Rx Var 11 : xpcethercatlib/EtherCAT PDO Receive  Priority=2  sig_name=Box 2 (ATRIAS 2.1 Leg (Medulla 1.5)).Power.Motor Voltage  sig_offset=1152  sig_type=uint16  type_size=16  sig_dim=1  device_id=0  sample_time=0.000500
  EtherCAT Rx Var 12 : xpcethercatlib/EtherCAT PDO Receive  Priority=2  sig_name=Box 2 (ATRIAS 2.1 Leg (Medulla 1.5)).Thermistors.Thermistor 0  sig_offset=1184  sig_type=uint16  type_size=16  sig_dim=1  device_id=0  sample_time=0.000500
  EtherCAT Rx Var 13 : xpcethercatlib/EtherCAT PDO Receive  Priority=2  sig_name=Box 2 (ATRIAS 2.1 Leg (Medulla 1.5)).Thermistors.Thermistor 1  sig_offset=1200  sig_type=uint16  type_size=16  sig_dim=1  device_id=0  sample_time=0.000500
  EtherCAT Rx Var 14 : xpcethercatlib/EtherCAT PDO Receive  Priority=2  sig_name=Box 2 (ATRIAS 2.1 Leg (Medulla 1.5)).Thermistors.Thermistor 2  sig_offset=1216  sig_type=uint16  type_size=16  sig_dim=1  device_id=0  sample_time=0.000500
  EtherCAT Rx Var 15 : xpcethercatlib/EtherCAT PDO Receive  Priority=2  sig_name=Box 2 (ATRIAS 2.1 Leg (Medulla 1.5)).Thermistors.Thermistor 3  sig_offset=1232  sig_type=uint16  type_size=16  sig_dim=1  device_id=0  sample_time=0.000500
  EtherCAT Rx Var 16 : xpcethercatlib/EtherCAT PDO Receive  Priority=2  sig_name=Box 2 (ATRIAS 2.1 Leg (Medulla 1.5)).Thermistors.Thermistor 4  sig_offset=1248  sig_type=uint16  type_size=16  sig_dim=1  device_id=0  sample_time=0.000500
  EtherCAT Rx Var 17 : xpcethercatlib/EtherCAT PDO Receive  Priority=2  sig_name=Box 2 (ATRIAS 2.1 Leg (Medulla 1.5)).Thermistors.Thermistor 5  sig_offset=1264  sig_type=uint16  type_size=16  sig_dim=1  device_id=0  sample_time=0.000500
  EtherCAT Rx Var 18 : xpcethercatlib/EtherCAT PDO Receive  Priority=2  sig_name=Box 2 (ATRIAS 2.1 Leg (Medulla 1.5)).uController Status.Counter  sig_offset=984  sig_type=uint8  type_size=8  sig_dim=1  device_id=0  sample_time=0.000500
  EtherCAT Rx Var 19 : xpcethercatlib/EtherCAT PDO Receive  Priority=2  sig_name=Box 2 (ATRIAS 2.1 Leg (Medulla 1.5)).uController Status.Error Flags  sig_offset=992  sig_type=uint8  type_size=8  sig_dim=1  device_id=0  sample_time=0.000500
  EtherCAT Rx Var 2 : xpcethercatlib/EtherCAT PDO Receive  Priority=2  sig_name=Box 2 (ATRIAS 2.1 Leg (Medulla 1.5)).Knee Force.Knee Force 1  sig_offset=1312  sig_type=uint16  type_size=16  sig_dim=1  device_id=0  sample_time=0.000500
  EtherCAT Rx Var 20 : xpcethercatlib/EtherCAT PDO Receive  Priority=2  sig_name=Box 2 (ATRIAS 2.1 Leg (Medulla 1.5)).uController Status.ID  sig_offset=968  sig_type=uint8  type_size=8  sig_dim=1  device_id=0  sample_time=0.000500
  EtherCAT Rx Var 21 : xpcethercatlib/EtherCAT PDO Receive  Priority=2  sig_name=Box 2 (ATRIAS 2.1 Leg (Medulla 1.5)).uController Status.Limit Switch  sig_offset=1000  sig_type=uint8  type_size=8  sig_dim=1  device_id=0  sample_time=0.000500
  EtherCAT Rx Var 22 : xpcethercatlib/EtherCAT PDO Receive  Priority=2  sig_name=Box 2 (ATRIAS 2.1 Leg (Medulla 1.5)).uController Status.State  sig_offset=976  sig_type=uint8  type_size=8  sig_dim=1  device_id=0  sample_time=0.000500
  EtherCAT Rx Var 23 : xpcethercatlib/EtherCAT PDO Receive  Priority=2  sig_name=Box 2 (ATRIAS 2.1 Leg (Medulla 1.5)).uController Status.Toe Sensor  sig_offset=1008  sig_type=uint16  type_size=16  sig_dim=1  device_id=0  sample_time=0.000500
  EtherCAT Rx Var 3 : xpcethercatlib/EtherCAT PDO Receive  Priority=2  sig_name=Box 2 (ATRIAS 2.1 Leg (Medulla 1.5)).Knee Force.Knee Force 2  sig_offset=1328  sig_type=uint16  type_size=16  sig_dim=1  device_id=0  sample_time=0.000500
  EtherCAT Rx Var 4 : xpcethercatlib/EtherCAT PDO Receive  Priority=2  sig_name=Box 2 (ATRIAS 2.1 Leg (Medulla 1.5)).Leg Encoder.Leg Encoder  sig_offset=1072  sig_type=uint32  type_size=32  sig_dim=1  device_id=0  sample_time=0.000500
  EtherCAT Rx Var 5 : xpcethercatlib/EtherCAT PDO Receive  Priority=2  sig_name=Box 2 (ATRIAS 2.1 Leg (Medulla 1.5)).Leg Encoder.Leg Encoder Timestamp  sig_offset=1104  sig_type=uint16  type_size=16  sig_dim=1  device_id=0  sample_time=0.000500
  EtherCAT Rx Var 6 : xpcethercatlib/EtherCAT PDO Receive  Priority=2  sig_name=Box 2 (ATRIAS 2.1 Leg (Medulla 1.5)).Measured Current.Amp 1 Measured Current  sig_offset=1280  sig_type=int16  type_size=16  sig_dim=1  device_id=0  sample_time=0.000500
  EtherCAT Rx Var 7 : xpcethercatlib/EtherCAT PDO Receive  Priority=2  sig_name=Box 2 (ATRIAS 2.1 Leg (Medulla 1.5)).Measured Current.Amp 2 Measured Current  sig_offset=1296  sig_type=int16  type_size=16  sig_dim=1  device_id=0  sample_time=0.000500
  EtherCAT Rx Var 8 : xpcethercatlib/EtherCAT PDO Receive  Priority=2  sig_name=Box 2 (ATRIAS 2.1 Leg (Medulla 1.5)).Motor Encoder.Motor Encoder  sig_offset=1024  sig_type=uint32  type_size=32  sig_dim=1  device_id=0  sample_time=0.000500
  EtherCAT Rx Var 9 : xpcethercatlib/EtherCAT PDO Receive  Priority=2  sig_name=Box 2 (ATRIAS 2.1 Leg (Medulla 1.5)).Motor Encoder.Motor Encoder Timestamp  sig_offset=1056  sig_type=uint16  type_size=16  sig_dim=1  device_id=0  sample_time=0.000500
  EtherCAT Tx Var 3 : xpcethercatlib/EtherCAT PDO Transmit   Priority=3  sig_name=Box 2 (ATRIAS 2.1 Leg (Medulla 1.5)).uControllerInput.Command  sig_offset=968  sig_type=uint8  type_size=8  sig_dim=1  device_id=0  sample_time=0.000500
  EtherCAT Tx Var 4 : xpcethercatlib/EtherCAT PDO Transmit   Priority=3  sig_name=Box 2 (ATRIAS 2.1 Leg (Medulla 1.5)).uControllerInput.Counter  sig_offset=976  sig_type=uint16  type_size=16  sig_dim=1  device_id=0  sample_time=0.000500
  EtherCAT Tx Var 5 : xpcethercatlib/EtherCAT PDO Transmit   Priority=3  sig_name=Box 2 (ATRIAS 2.1 Leg (Medulla 1.5)).uControllerInput.Motor Current  sig_offset=992  sig_type=int32  type_size=32  sig_dim=1  device_id=0  sample_time=0.000500
  Mux1 : Mux  Inputs=2
  Mux2 : Mux  Inputs=2
  Mux5 : Mux  Inputs=6
  LegEncoder : Outport
  MotorEncoder : Outport  Port=2
  ToeSensor : Outport  Port=3
  LimitSwitch : Outport  Port=4
  ID : Outport  Port=5
  State : Outport  Port=6
  Counter : Outport  Port=7
  ErrorFlags : Outport  Port=8
  IncEncoder : Outport  Port=9
  LegEncoderTimestamp : Outport  Port=10
  MotorEncoderTimestamp : Outport  Port=11
  IncEncoderTimestamp : Outport  Port=12
  MotorVoltage : Outport  Port=13
  LogicVoltage : Outport  Port=14
  Thermistors : Outport  Port=15
  AmpMeasuredCurrent : Outport  Port=16
  KneeForce : Outport  Port=17
  wires:
  Data Type Conversion3/1 -> EtherCAT Tx Var 3/1
  Data Type Conversion4/1 -> EtherCAT Tx Var 4/1
  Data Type Conversion5/1 -> EtherCAT Tx Var 5/1
  "EtherCAT Rx Var "/1 -> IncEncoder/1
  EtherCAT Rx Var 1/1 -> IncEncoderTimestamp/1
  EtherCAT Rx Var 2/1 -> Mux2/1
  EtherCAT Rx Var 3/1 -> Mux2/2
  EtherCAT Rx Var 4/1 -> LegEncoder/1
  EtherCAT Rx Var 5/1 -> LegEncoderTimestamp/1
  EtherCAT Rx Var 6/1 -> Mux1/1
  EtherCAT Rx Var 7/1 -> Mux1/2
  EtherCAT Rx Var 8/1 -> MotorEncoder/1
  EtherCAT Rx Var 9/1 -> MotorEncoderTimestamp/1
  EtherCAT Rx Var 10/1 -> LogicVoltage/1
  EtherCAT Rx Var 11/1 -> MotorVoltage/1
  EtherCAT Rx Var 12/1 -> Mux5/1
  EtherCAT Rx Var 13/1 -> Mux5/2
  EtherCAT Rx Var 14/1 -> Mux5/3
  EtherCAT Rx Var 15/1 -> Mux5/4
  EtherCAT Rx Var 16/1 -> Mux5/5
  EtherCAT Rx Var 17/1 -> Mux5/6
  EtherCAT Rx Var 18/1 -> Counter/1
  EtherCAT Rx Var 19/1 -> ErrorFlags/1
  EtherCAT Rx Var 20/1 -> ID/1
  EtherCAT Rx Var 21/1 -> LimitSwitch/1
  EtherCAT Rx Var 22/1 -> State/1
  EtherCAT Rx Var 23/1 -> ToeSensor/1
  MedullaCmd/1 -> Data Type Conversion3/1
  MedullaCounter/1 -> Data Type Conversion4/1
  MotorCmd/1 -> Data Type Conversion5/1
  Mux5/1 -> Thermistors/1
  Mux1/1 -> AmpMeasuredCurrent/1
  Mux2/1 -> KneeForce/1
